simulink model "ECU_Auxiliaries_Signal_Coordinator"  (R2016b)
settings: Solver=FixedStepDiscrete  StartTime=0.0  StopTime=inf  FixedStep=ECUAuxSigCoorr.tiSimnTiStep_C.Value  RelTol=1e-3  EnableMultiTasking=on
settings Model: Creator=djuenema  LastModifiedBy=djuenema
settings DataIOCC: SaveFormat=StructureWithTime  SaveOutput=off  DSMLogging=off  VisualizeSimOutput=off  SaveTime=off  SignalLoggingName=Results
settings OptimizationCC: BlockReduction=off  ConditionallyExecuteInputs=off  LifeSpan=inf
settings DebuggingCC: AllowSymbolicDim=off  SFUnexpectedBacktrackingDiag=warning  SFNoUnconditionalDefaultTransitionDiag=warning  SFExecutionAtInitializationDiag=none
settings ModelReferenceCC: ModelReferenceNumInstancesAllowed=Single  PropagateSignalLabelsOutOfModel=off
settings GRTTargetCC: TargetLangStandard=C89/C90 (ANSI)
settings ConfigComp: CovMetricSettings=dw  CovHtmlReporting=on  CovSaveCumulativeToWorkspaceVar=on  CovSaveSingleToWorkspaceVar=on  CovExternalEMLEnable=off

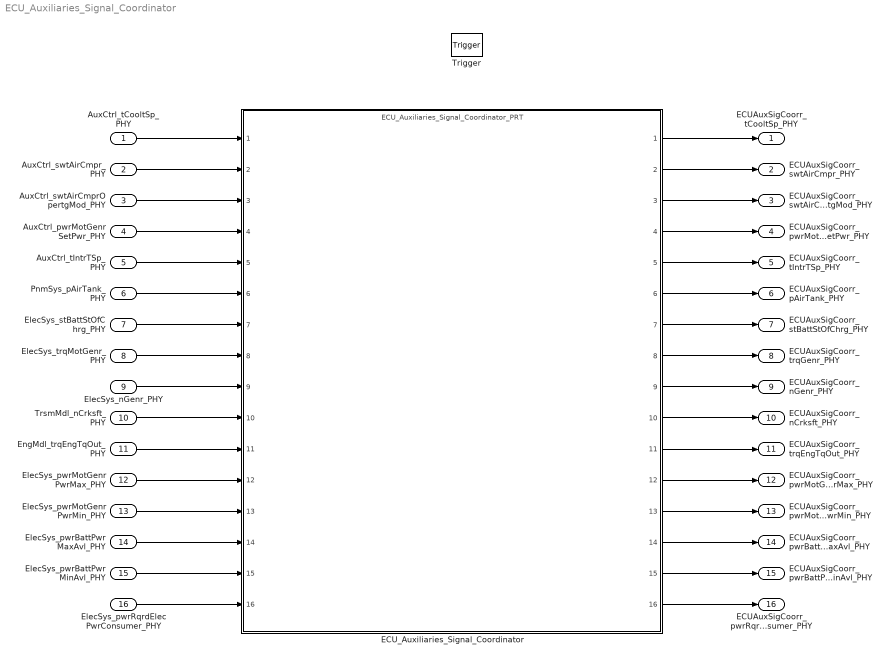
== system ECU_Auxiliaries_Signal_Coordinator ==
  AuxCtrl_tCooltSp_PHY : Inport
  AuxCtrl_swtAirCmpr_PHY : Inport  Port=2
  AuxCtrl_swtAirCmprOpertgMod_PHY : Inport  Port=3
  AuxCtrl_pwrMotGenrSetPwr_PHY : Inport  Port=4
  AuxCtrl_tIntrTSp_PHY : Inport  Port=5
  PnmSys_pAirTank_PHY : Inport  Port=6
  ElecSys_stBattStOfChrg_PHY : Inport  Port=7
  ElecSys_trqMotGenr_PHY : Inport  Port=8
  ElecSys_nGenr_PHY : Inport  Port=9
  TrsmMdl_nCrksft_PHY : Inport  Port=10
  EngMdl_trqEngTqOut_PHY : Inport  Port=11
  ElecSys_pwrMotGenrPwrMax_PHY : Inport  Port=12
  ElecSys_pwrMotGenrPwrMin_PHY : Inport  Port=13
  ElecSys_pwrBattPwrMaxAvl_PHY : Inport  Port=14
  ElecSys_pwrBattPwrMinAvl_PHY : Inport  Port=15
  ElecSys_pwrRqrdElecPwrConsumer_PHY : Inport  Port=16
  Trigger : TriggerPort  TriggerType=function-call  VariantControl=Variant  PortDimensions=1
  ECU_Auxiliaries_Signal_Coordinator : ModelReference  ModelNameDialog=ECU_Auxiliaries_Signal_Coordinator_PRT  ModelReferenceVersion=1.3  CopyOfModelProtected=on
  ECUAuxSigCoorr_tCooltSp_PHY : Outport
  ECUAuxSigCoorr_swtAirCmpr_PHY : Outport  Port=2
  ECUAuxSigCoorr_swtAirCmprOpertgMod_PHY : Outport  Port=3
  ECUAuxSigCoorr_pwrMotGenrSetPwr_PHY : Outport  Port=4
  ECUAuxSigCoorr_tIntrTSp_PHY : Outport  Port=5
  ECUAuxSigCoorr_pAirTank_PHY : Outport  Port=6
  ECUAuxSigCoorr_stBattStOfChrg_PHY : Outport  Port=7
  ECUAuxSigCoorr_trqGenr_PHY : Outport  Port=8
  ECUAuxSigCoorr_nGenr_PHY : Outport  Port=9
  ECUAuxSigCoorr_nCrksft_PHY : Outport  Port=10
  ECUAuxSigCoorr_trqEngTqOut_PHY : Outport  Port=11
  ECUAuxSigCoorr_pwrMotGenrPwrMax_PHY : Outport  Port=12
  ECUAuxSigCoorr_pwrMotGenrPwrMin_PHY : Outport  Port=13
  ECUAuxSigCoorr_pwrBattPwrMaxAvl_PHY : Outport  Port=14
  ECUAuxSigCoorr_pwrBattPwrMinAvl_PHY : Outport  Port=15
  ECUAuxSigCoorr_pwrRqrdElecPwrConsumer_PHY : Outport  Port=16
  wires:
  AuxCtrl_swtAirCmprOpertgMod_PHY/1 -> ECU_Auxiliaries_Signal_Coordinator/3
  AuxCtrl_tCooltSp_PHY/1 -> ECU_Auxiliaries_Signal_Coordinator/1
  AuxCtrl_swtAirCmpr_PHY/1 -> ECU_Auxiliaries_Signal_Coordinator/2
  ECU_Auxiliaries_Signal_Coordinator/1 -> ECUAuxSigCoorr_tCooltSp_PHY/1
  PnmSys_pAirTank_PHY/1 -> ECU_Auxiliaries_Signal_Coordinator/6
  AuxCtrl_tIntrTSp_PHY/1 -> ECU_Auxiliaries_Signal_Coordinator/5
  AuxCtrl_pwrMotGenrSetPwr_PHY/1 -> ECU_Auxiliaries_Signal_Coordinator/4
  ElecSys_stBattStOfChrg_PHY/1 -> ECU_Auxiliaries_Signal_Coordinator/7
  ElecSys_nGenr_PHY/1 -> ECU_Auxiliaries_Signal_Coordinator/9
  ElecSys_trqMotGenr_PHY/1 -> ECU_Auxiliaries_Signal_Coordinator/8
  ECU_Auxiliaries_Signal_Coordinator/7 -> ECUAuxSigCoorr_stBattStOfChrg_PHY/1
  ECU_Auxiliaries_Signal_Coordinator/6 -> ECUAuxSigCoorr_pAirTank_PHY/1
  ECU_Auxiliaries_Signal_Coordinator/5 -> ECUAuxSigCoorr_tIntrTSp_PHY/1
  ECU_Auxiliaries_Signal_Coordinator/4 -> ECUAuxSigCoorr_pwrMotGenrSetPwr_PHY/1
  ECU_Auxiliaries_Signal_Coordinator/3 -> ECUAuxSigCoorr_swtAirCmprOpertgMod_PHY/1
  ECU_Auxiliaries_Signal_Coordinator/2 -> ECUAuxSigCoorr_swtAirCmpr_PHY/1
  ECU_Auxiliaries_Signal_Coordinator/9 -> ECUAuxSigCoorr_nGenr_PHY/1
  ECU_Auxiliaries_Signal_Coordinator/8 -> ECUAuxSigCoorr_trqGenr_PHY/1
  ElecSys_pwrRqrdElecPwrConsumer_PHY/1 -> ECU_Auxiliaries_Signal_Coordinator/16
  ElecSys_pwrBattPwrMinAvl_PHY/1 -> ECU_Auxiliaries_Signal_Coordinator/15
  ElecSys_pwrMotGenrPwrMin_PHY/1 -> ECU_Auxiliaries_Signal_Coordinator/13
  ElecSys_pwrBattPwrMaxAvl_PHY/1 -> ECU_Auxiliaries_Signal_Coordinator/14
  TrsmMdl_nCrksft_PHY/1 -> ECU_Auxiliaries_Signal_Coordinator/10
  ElecSys_pwrMotGenrPwrMax_PHY/1 -> ECU_Auxiliaries_Signal_Coordinator/12
  EngMdl_trqEngTqOut_PHY/1 -> ECU_Auxiliaries_Signal_Coordinator/11
  ECU_Auxiliaries_Signal_Coordinator/14 -> ECUAuxSigCoorr_pwrBattPwrMaxAvl_PHY/1
  ECU_Auxiliaries_Signal_Coordinator/13 -> ECUAuxSigCoorr_pwrMotGenrPwrMin_PHY/1
  ECU_Auxiliaries_Signal_Coordinator/12 -> ECUAuxSigCoorr_pwrMotGenrPwrMax_PHY/1
  ECU_Auxiliaries_Signal_Coordinator/11 -> ECUAuxSigCoorr_trqEngTqOut_PHY/1
  ECU_Auxiliaries_Signal_Coordinator/16 -> ECUAuxSigCoorr_pwrRqrdElecPwrConsumer_PHY/1
  ECU_Auxiliaries_Signal_Coordinator/15 -> ECUAuxSigCoorr_pwrBattPwrMinAvl_PHY/1
  ECU_Auxiliaries_Signal_Coordinator/10 -> ECUAuxSigCoorr_nCrksft_PHY/1
